simulink model "AFPIDC_PCT100"  (R2021a)
settings: Solver=VariableStepAuto  StartTime=0.0  StopTime=15.1010  RelTol=1e-3
undefined symbols (not defined in the file or in its folder): dE_kd, dE_ki, dE_kp, DiscIntNeverNeededParam, E_kd, E_ki, E_kp, U_kd, U_ki, U_kp
libraries: simulink x4, pid_lib x1
settings Model: Creator=ASUS  LastModifiedBy=ASUS

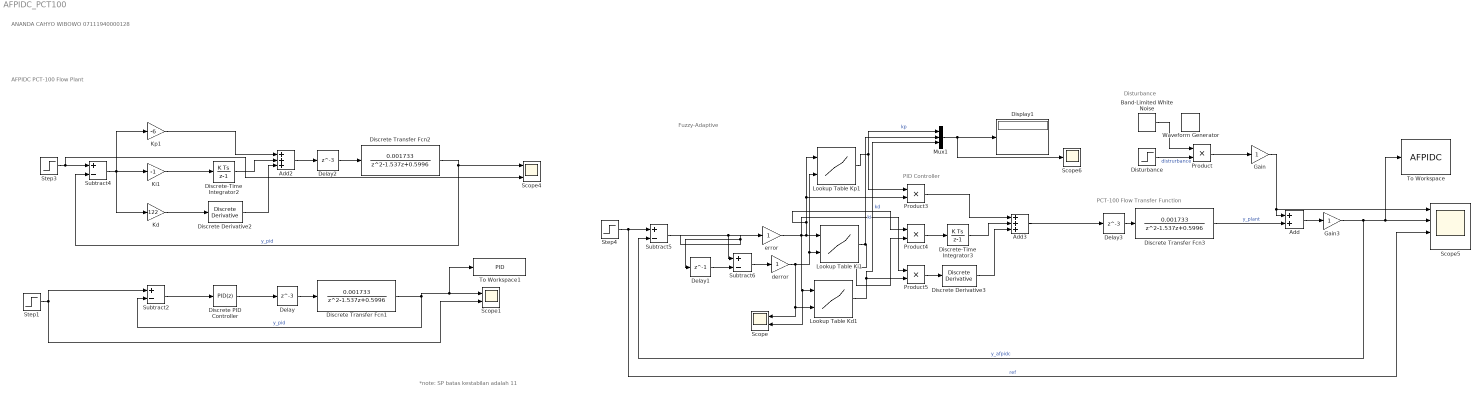
== system AFPIDC_PCT100 ==
  note: *note: SP batas kestabilan adalah 11
  note: PCT-100 Flow Transfer Function
  note: PID Controller
  note: Fuzzy-Adaptive
  note: Disturbance
  note: AFPIDC PCT-100 Flow Plant
  note: ANANDA CAHYO WIBOWO
      | 07111940000128
  Add : Sum
  Add2 : Sum  Inputs=+++
  Add3 : Sum  Inputs=+++
  Band-Limited White Noise : simulink/Sources/Band-Limited White Noise  Cov=[10e-4]  Ts=0.1  seed=[10e2]
  Delay : Delay  DelayLength=3  SampleTime=0.1
  Delay1 : Delay  DelayLength=1  SampleTime=0.1
  Delay2 : Delay  DelayLength=3  SampleTime=0.1
  Delay3 : Delay  DelayLength=3  SampleTime=0.1
  Discrete Transfer Fcn1 : DiscreteTransferFcn  Numerator=[0.001733]  Denominator=[1 -1.537 0.5996]  SampleTime=0.1
  Discrete Transfer Fcn2 : DiscreteTransferFcn  Numerator=[0.001733]  Denominator=[1 -1.537 0.5996]  SampleTime=0.1
  Discrete Transfer Fcn3 : DiscreteTransferFcn  Numerator=[0.001733]  Denominator=[1 -1.537 0.5996]  SampleTime=0.1
  Discrete Derivative2 : simulink/Discrete/Discrete Derivative  gainval=1.0  ICPrevScaledInput=0.0  OutMin=[]  OutMax=[]  OutDataType=fixdt(1, 16)  OutScaling=2^-10  DoSatur=off
  Discrete Derivative3 : simulink/Discrete/Discrete Derivative  gainval=1.0  ICPrevScaledInput=0.0  OutMin=[]  OutMax=[]  OutDataType=fixdt(1, 16)  OutScaling=2^-10  DoSatur=off
  Discrete PID Controller : pid_lib/PID Controller  Controller=PID  Form=Parallel  TimeDomain=Discrete-time  UseExternalTs=off  SampleTime=0.1  IntegratorMethod=Forward Euler  FilterMethod=Forward Euler  ControllerParametersSource=internal  P=6.0006084220144  I=20.5044954290519  D=0  UseFilter=on  N=100  TunerSelectOption=Transfer Function Based (PID Tuner App)  InitialConditionSource=internal  InitialConditionForIntegrator=0  InitialConditionForFilter=0  DifferentiatorICPrevScaledInput=0  ExternalReset=none  TrackingMode=off  Kt=1  LimitOutput=off  SatLimitsSource=internal  UpperSaturationLimit=inf  LowerSaturationLimit=-inf  LinearizeAsGain=off  AntiWindupMode=none  Kb=1  POutMin=[]  POutMax=[]  IOutMin=[]  IOutMax=[]  DOutMin=[]  DOutMax=[]  NOutMin=[]  NOutMax=[]  SumOutMin=[]  SumOutMax=[]  SaturationOutMin=[]  SaturationOutMax=[]  PParamMin=[]  PParamMax=[]  IParamMin=[]  IParamMax=[]  DParamMin=[]  DParamMax=[]  NParamMin=[]  NParamMax=[]  KbParamMin=[]  KbParamMax=[]  KtParamMin=[]  KtParamMax=[]  KbOutMin=[]  KbOutMax=[]  KtOutMin=[]  KtOutMax=[]  IntegratorOutMin=[]  IntegratorOutMax=[]  FilterOutMin=[]  FilterOutMax=[]  SumI1OutMin=[]  SumI1OutMax=[]  SumI2OutMin=[]  SumI2OutMax=[]  SumI3OutMin=[]  SumI3OutMax=[]  SumI4OutMin=[]  SumI4OutMax=[]  SumDOutMin=[]  SumDOutMax=[]  DifferentiatorOutMin=[]  DifferentiatorOutMax=[]  FilterDiffOutCoefMin=[]  FilterDiffOutCoefMax=[]  ReciprocalOutMin=[]  ReciprocalOutMax=[]  SumDenOutMin=[]  SumDenOutMax=[]  SumNumOutMin=[]  SumNumOutMax=[]  DivideOutMin=[]  DivideOutMax=[]  UdiffTsProdOutMin=[]  UdiffTsProdOutMax=[]  NTsProdOutMin=[]  NTsProdOutMax=[]  UintegralTsProdOutMin=[]  UintegralTsProdOutMax=[]  UngainTsProdOutMin=[]  UngainTsProdOutMax=[]  IntegratorContinuousStateAttributes=''  IntegratorStateMustResolveToSignalObject=off  IntegratorRTWStateStorageClass=Auto  FilterContinuousStateAttributes=''  FilterStateMustResolveToSignalObject=off  FilterRTWStateStorageClass=Auto  ParallelPVariant=InternalParameters  IdealPVariant=Disabled  IVariant=InternalParameters  DVariant=InternalParameters  IntegratorVariant=Discrete  SatVariant=Disabled  AWVariant=Passthrough  PCopyVariant=Disabled  TRVariant=Disabled  FdbkBlocksVariant=Forward  IdealPFdbkVariant=Disabled  SatFdbkVariant=Disabled  DerivativeFilterVariant=ForwardEulerFilter  NVariant=InternalParameters  NCopyVariant=Disabled  FilterICVariant=InternalICsFilter  IntegratorICVariant=InternalICs  ExternalResetVariant=Disabled  TRSumVariant=Passthrough  SumFdbkVariant=Disabled  SumVariant=Sum_PID  TsampFilterVariant=InternalTs  TsampNgainVariant=Passthrough  TsampIntegralVariant=Passthrough  ExternalSaturationOutDataTypeStr=Inherit: Same as second input
  Discrete-Time Integrator2 : DiscreteIntegrator  SampleTime=0.1  ICPrevOutput=DiscIntNeverNeededParam  ICPrevScaledInput=DiscIntNeverNeededParam
  Discrete-Time Integrator3 : DiscreteIntegrator  SampleTime=0.1  ICPrevOutput=DiscIntNeverNeededParam  ICPrevScaledInput=DiscIntNeverNeededParam
  Display1 : Display
  Disturbance : Step  Time=0  After=0.5  SampleTime=0
  Gain : Gain
  Gain3 : Gain
  Kd : Gain  Gain=122
  Ki1 : Gain  Gain=-1
  Kp1 : Gain  Gain=-6
  Lookup Table Kd1 : Lookup_n-D  BreakpointsForDimension1=E_kd(1,:)  BreakpointsForDimension2=dE_kd(:,1)  Table=U_kd  InternalRulePriority=Speed  RndMeth=Simplest  InputSameDT=on
      settings: InputPortMap=u0,u1
  Lookup Table Ki1 : Lookup_n-D  BreakpointsForDimension1=E_ki(1,:)  BreakpointsForDimension2=dE_ki(:,1)  Table=U_ki  InternalRulePriority=Speed  RndMeth=Simplest  InputSameDT=on
      settings: InputPortMap=u0,u1
  Lookup Table Kp1 : Lookup_n-D  BreakpointsForDimension1=E_kp(1,:)  BreakpointsForDimension2=dE_kp(:,1)  Table=U_kp  InternalRulePriority=Speed  RndMeth=Simplest  InputSameDT=on
      settings: InputPortMap=u0,u1
  Mux1 : Mux  Inputs=3
  Product{,3..5} (4 alike) : Product
  Scope : Scope  NumInputPorts=2
  Scope1 : Scope  NumInputPorts=2
  Scope4 : Scope  NumInputPorts=3
  Scope5 : Scope  NumInputPorts=4
  Scope6 : Scope
  Step1 : Step  SampleTime=0.1
  Step3 : Step  SampleTime=0.1
  Step4 : Step  SampleTime=0.1
  Subtract{2,4..6} (4 alike) : Sum  Inputs=+-
  To Workspace : ToWorkspace  VariableName=AFPIDC  SaveFormat=Timeseries  SampleTime=0.1
  To Workspace1 : ToWorkspace  VariableName=PID  SaveFormat=Timeseries  SampleTime=0.1
  Waveform Generator : simulink/Sources/Waveform Generator  OutMin=[]  OutMax=[]  OutDataTypeStr=double  SelectedSignal=1  Signals=sin(0.2,2*pi,0) + sin(0.3,0.5*pi,pi/2)  BlockNames=MultiportSwitch_ae95b8f8bdf8464  SampleTime=0.1
  derror : Gain
  error : Gain
  wires:
  Lookup Table Kd1/1 -> Mux1/3, Product5/2  "kd"
  Discrete Transfer Fcn3/1 -> Add/2  "y_plant"
  Discrete-Time Integrator3/1 -> Add3/2
  Discrete Derivative3/1 -> Add3/3
  Step1/1 -> Scope1/2, Subtract2/1
  Discrete PID Controller/1 -> Delay/1
  Subtract5/1 -> Subtract6/1, error/1, Delay1/1
  Product5/1 -> Discrete Derivative3/1
  Kp1/1 -> Add2/1
  Delay1/1 -> Subtract6/2
  Discrete-Time Integrator2/1 -> Add2/2
  Ki1/1 -> Discrete-Time Integrator2/1
  Subtract2/1 -> Discrete PID Controller/1
  derror/1 -> Scope/1, Lookup Table Kd1/2, Lookup Table Ki1/2, Lookup Table Kp1/2
  Step3/1 -> Scope4/3, Subtract4/1
  Discrete Transfer Fcn1/1 -> Subtract2/2, To Workspace1/1, Scope1/1  "y_pid"
  Lookup Table Ki1/1 -> Mux1/2, Product4/2  "ki"
  error/1 -> Scope/2, Lookup Table Kd1/1, Product5/1, Lookup Table Ki1/1, Product4/1, Product3/2, Lookup Table Kp1/1
  Step4/1 -> Scope5/3, Subtract5/1  "ref"
  Product4/1 -> Discrete-Time Integrator3/1
  Lookup Table Kp1/1 -> Mux1/1, Product3/1  "kp"
  Discrete Derivative2/1 -> Add2/3
  Mux1/1 -> Scope6/1, Display1/1
  Kd/1 -> Discrete Derivative2/1
  Gain3/1 -> Subtract5/2, To Workspace/1, Scope5/2  "y_afpidc"
  Product3/1 -> Add3/1
  Subtract6/1 -> derror/1
  Subtract4/1 -> Kd/1, Ki1/1, Kp1/1
  Add/1 -> Gain3/1
  Delay/1 -> Discrete Transfer Fcn1/1
  Add2/1 -> Delay2/1
  Delay2/1 -> Discrete Transfer Fcn2/1
  Discrete Transfer Fcn2/1 -> Scope4/1, Subtract4/2  "y_pid"
  Add3/1 -> Delay3/1
  Delay3/1 -> Discrete Transfer Fcn3/1
  Gain/1 -> Scope5/1, Add/1
  Disturbance/1 -> Product/2  "distrurbance"
  Product/1 -> Gain/1
  Band-Limited White Noise/1 -> Product/1
